simulink model "LOTKAVOLTERRA"  (R2023a)
settings: Solver=FixedStepAuto  StartTime=0.0  StopTime=100  FixedStep=0.1  MaxStep=2.0  RelTol=1e-3
settings Model: Creator=Lenovo  LastModifiedBy=Lenovo
settings DataIOCC: InspectSignalLogs=on  ReturnWorkspaceOutputs=off  TimeSaveName=t

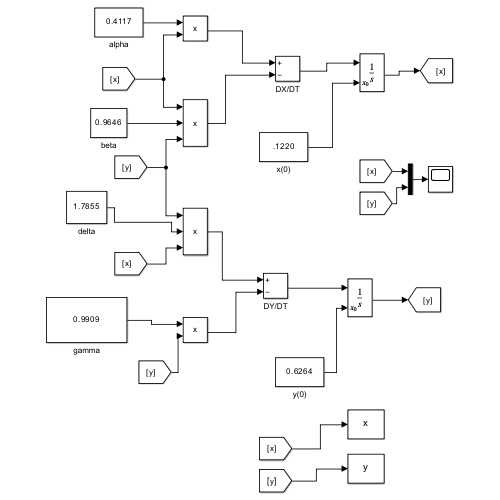
[thumbnail: Simulink's stored preview of the top-level diagram]
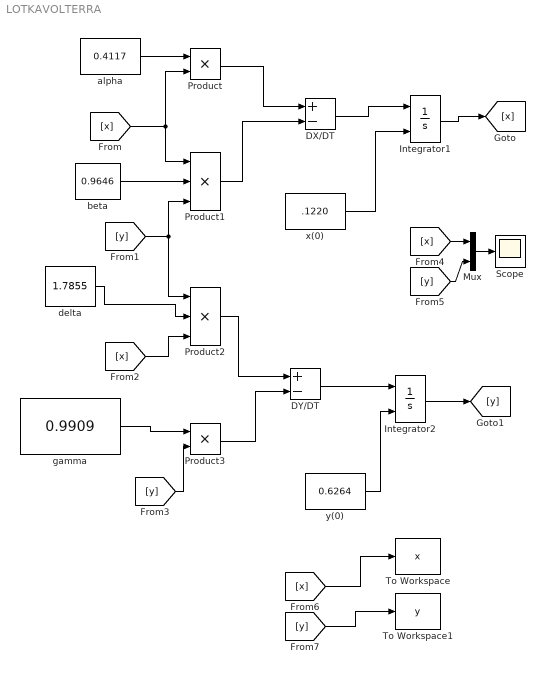
== system LOTKAVOLTERRA ==
  DX/DT : Sum  Inputs=+-
  DY/DT : Sum  Inputs=+-
  Integrator1 : Integrator  InitialConditionSource=external
  Integrator2 : Integrator  InitialConditionSource=external
  Mux : Mux  Inputs=2
  Product : Product
  Product1 : Product  Inputs=3
  Product2 : Product  Inputs=3
  Product3 : Product
  Scope : Scope
  To Workspace : ToWorkspace  VariableName=x  SampleTime=-1
  To Workspace1 : ToWorkspace  VariableName=y  SampleTime=-1
  alpha : Constant  Value=0.4117
  beta : Constant  Value=0.9646
  delta : Constant  Value=1.7855
  gamma : Constant  Value=0.9909
  x(0) : Constant  Value=.1220
  y(0) : Constant  Value=0.6264
  wires:
  alpha/1 -> Product/1
  [x] -> Product1/1, Product/2
  beta/1 -> Product1/2
  [y] -> Product2/1, Product1/3
  delta/1 -> Product2/2
  [x] -> Product2/3
  gamma/1 -> Product3/1
  [y] -> Product3/2
  Product3/1 -> DY/DT/2
  Product2/1 -> DY/DT/1
  Product/1 -> DX/DT/1
  Product1/1 -> DX/DT/2
  Integrator1/1 -> [x]
  DX/DT/1 -> Integrator1/1
  x(0)/1 -> Integrator1/2
  DY/DT/1 -> Integrator2/1
  y(0)/1 -> Integrator2/2
  Integrator2/1 -> [y]
  Mux/1 -> Scope/1
  [y] -> Mux/2
  [x] -> Mux/1
  [x] -> To Workspace/1
  [y] -> To Workspace1/1
